simulink model "trial1"  (R2024a)
settings: Solver=VariableStepAuto  StartTime=0.0  StopTime=20  RelTol=1e-3

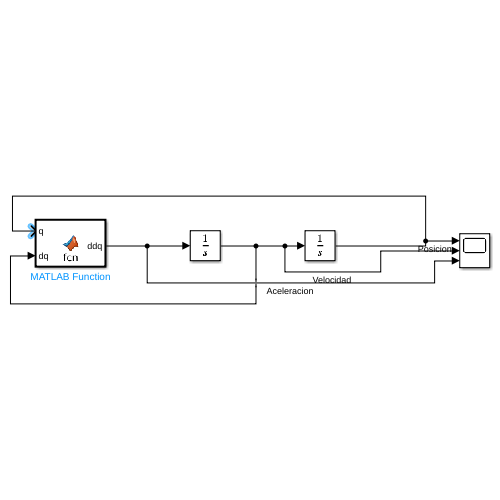
[thumbnail: Simulink's stored preview of the top-level diagram]
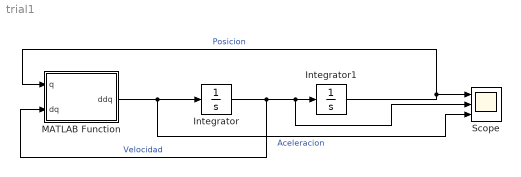
== system trial1 ==
  Integrator : Integrator
  Integrator1 : Integrator
  MATLAB Function : MATLAB Function  TreatAsAtomicUnit=on
  Scope : Scope  NumInputPorts=3
  wires:
  MATLAB Function/1(ddq) -> Scope/3, Integrator/1  "Aceleracion"
  Integrator1/1 -> Scope/1, MATLAB Function/1(q)  "Posicion"
  Integrator/1 -> MATLAB Function/2(dq), Scope/2, Integrator1/1  "Velocidad"

== matlab function trial1/MATLAB Function ==
  data: q input; ddq output; dq input
function ddq = fcn(q, dq)

k=0.01;
m=0.75;
l=0.36
g=9.8
t=1

a = l/2
j = 4*(m*a*a)/3
ddq = (t - (m*g*a*cos(q)) - (k*dq))/j
